simulink model "PracticaUdeAII"  (R2018a)
settings: Solver=VariableStepAuto  StartTime=0.0  StopTime=tsim  RelTol=1e-3
values from neighbouring files (symbols this model uses):
  den1 = [tao 1]    [EjmModelos.m]
  den2 = [t1*t2 t1+t2 1]    [EjmModelos.m]
  num1 = K    [EjmModelos.m]
  num2 = K    [EjmModelos.m]
  timeHead1 = t63-tao    (= 368.5)    [EjmModelos.m]
  tm2 = 1.5552*t25 - 0.5552*t75    (= 113.6992)    [EjmModelos.m]
  tu = 1    [EjmModelos.m]
settings Model: Creator=USER  LastModifiedBy=USER

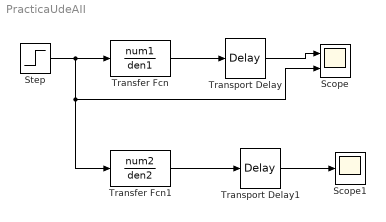
== system PracticaUdeAII ==
  Scope : Scope  NumInputPorts=2
  Scope1 : Scope
  Step : Step  Time=tu  After=5  SampleTime=0
  Transfer Fcn : TransferFcn  Numerator=num1  Denominator=den1
  Transfer Fcn1 : TransferFcn  Numerator=num2  Denominator=den2
  Transport Delay : TransportDelay  DelayTime=timeHead1
  Transport Delay1 : TransportDelay  DelayTime=tm2
  wires:
  Transfer Fcn/1 -> Transport Delay/1
  Transport Delay/1 -> Scope/1
  Step/1 -> Transfer Fcn1/1, Scope/2, Transfer Fcn/1
  Transport Delay1/1 -> Scope1/1
  Transfer Fcn1/1 -> Transport Delay1/1
